simulink model "Test3"  (R2013a)
settings: Solver=ode45  StartTime=0.0  StopTime=10e-3  MaxStep=1e-4  RelTol=1e-3
undefined symbols (not defined in the file or in its folder): Lc, Rc, Rsh
libraries: simulink x1
settings Model: Creator=mainster  LastModifiedBy=mainster

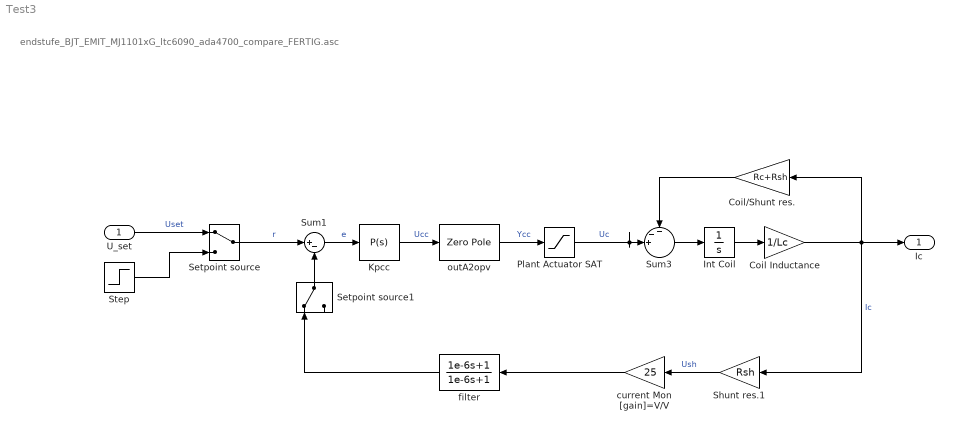
== system Test3 ==
  note: endstufe_BJT_EMIT_MJ1101xG_ltc6090_ada4700_compare_FERTIG.asc
  U_set : Inport
  Coil Inductance : Gain  Gain=1/Lc
  Coil/Shunt res. : Gain  Gain=Rc+Rsh
  Int Coil : Integrator
  Kpcc : simulink/Continuous/PID Controller  Controller=P  TimeDomain=Continuous-time  SampleTime=-1  IntegratorMethod=Forward Euler  FilterMethod=Forward Euler  Form=Ideal  P=4.5  I=14078.2261040339  D=0  N=100  InitialConditionSource=internal  InitialConditionForIntegrator=0  InitialConditionForFilter=0  ExternalReset=none  LimitOutput=off  UpperSaturationLimit=inf  LowerSaturationLimit=-inf  LinearizeAsGain=on  AntiWindupMode=none  Kb=1  TrackingMode=off  Kt=1  PParamMin=[]  PParamMax=[]  IParamMin=[]  IParamMax=[]  DParamMin=[]  DParamMax=[]  NParamMin=[]  NParamMax=[]  KbParamMin=[]  KbParamMax=[]  KtParamMin=[]  KtParamMax=[]  POutMin=[]  POutMax=[]  IOutMin=[]  IOutMax=[]  DOutMin=[]  DOutMax=[]  NOutMin=[]  NOutMax=[]  KbOutMin=[]  KbOutMax=[]  KtOutMin=[]  KtOutMax=[]  IntegratorOutMin=[]  IntegratorOutMax=[]  FilterOutMin=[]  FilterOutMax=[]  SumOutMin=[]  SumOutMax=[]  SumI1OutMin=[]  SumI1OutMax=[]  SumI2OutMin=[]  SumI2OutMax=[]  SumI3OutMin=[]  SumI3OutMax=[]  SumDOutMin=[]  SumDOutMax=[]  SaturationOutMin=[]  SaturationOutMax=[]  IntegratorContinuousStateAttributes=''  IntegratorStateMustResolveToSignalObject=off  IntegratorRTWStateStorageClass=Auto  FilterContinuousStateAttributes=''  FilterStateMustResolveToSignalObject=off  FilterRTWStateStorageClass=Auto
      settings: AttributesFormatString=Kp=%<P>
  Plant Actuator SAT : Saturate  UpperLimit=150  LowerLimit=-150
      settings: AttributesFormatString=U_lim=+-%<UpperLimit>V
  Setpoint source : ManualSwitch
  Setpoint source1 : ManualSwitch
  Shunt res.1 : Gain  Gain=Rsh
  Step : Step  SampleTime=0
  Sum1 : Sum  Inputs=|+-
  Sum3 : Sum  Inputs=--+||
  current Mon [gain]=V/V : Gain  Gain=25
  filter : TransferFcn  Numerator=[1e-6 1]  Denominator=[1e-6 1]
  outA2opv : ZeroPole  Zeros=3.4653e+08  Poles=-2.6678e+08  Gain=-0.7684
  Ic : Outport
  wires:
  outA2opv/1 -> Plant Actuator SAT/1  "Ycc"
  Sum1/1 -> Kpcc/1  "e"
  Coil Inductance/1 -> Ic/1, Shunt res.1/1, Coil/Shunt res./1  "Ic"
  Plant Actuator SAT/1 -> Sum3/3  "Uc"
  Coil/Shunt res./1 -> Sum3/1
  Sum3/1 -> Int Coil/1
  Int Coil/1 -> Coil Inductance/1
  Shunt res.1/1 -> current Mon [gain]=V/V/1  "Ush"
  current Mon [gain]=V/V/1 -> filter/1
  ? -> Sum3/2
  U_set/1 -> Setpoint source/1  "Uset"
  Step/1 -> Setpoint source/2
  Setpoint source/1 -> Sum1/1  "r"
  Kpcc/1 -> outA2opv/1  "Ucc"
  filter/1 -> Setpoint source1/1
  Setpoint source1/1 -> Sum1/2
